simulink model "Loop_Back_Testing"  (R2022a)
settings: Solver=FixedStepAuto  StartTime=0.0  StopTime=inf  FixedStep=.005  RelTol=1e-6
model workspace (MAT data in the model file):
  DEV_ID = 3
libraries: speedgoatlib_IO691 x5, canmsglib x4
settings Model: SimulationMode=external  ExtModeEnableFloating=off  Creator=celwe  LastModifiedBy=celwe
settings SolverCC: ConcurrentTasks=on  PositivePriorityOrder=on
settings OptimizationCC: BlockReduction=off  OptimizeBlockIOStorage=off
settings DebuggingCC: TasksWithSamePriorityMsg=none
settings HardwareCC: ProdBitPerLong=64  ProdLongLongMode=on  ProdHWDeviceType=Intel->x86-64 (Linux 64)
settings RTWCC: Description=Simulink Real-Time  SystemTargetFile=slrealtime.tlc  TemplateMakefile=slrealtime_default_tmf  Toolchain=Simulink Real-Time Toolchain  BuildConfiguration=Faster Runs  CodeExecutionProfiling=on  TargetLang=C++

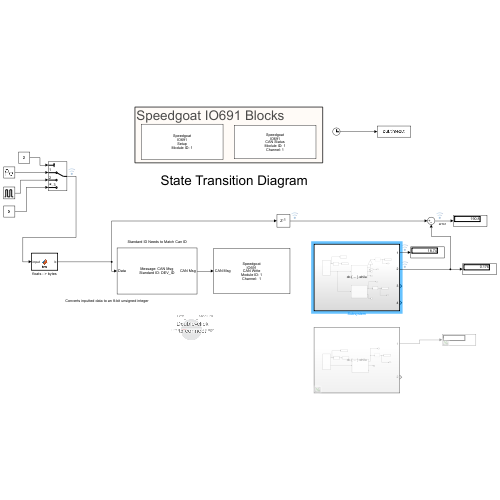
[thumbnail: Simulink's stored preview of the top-level diagram]
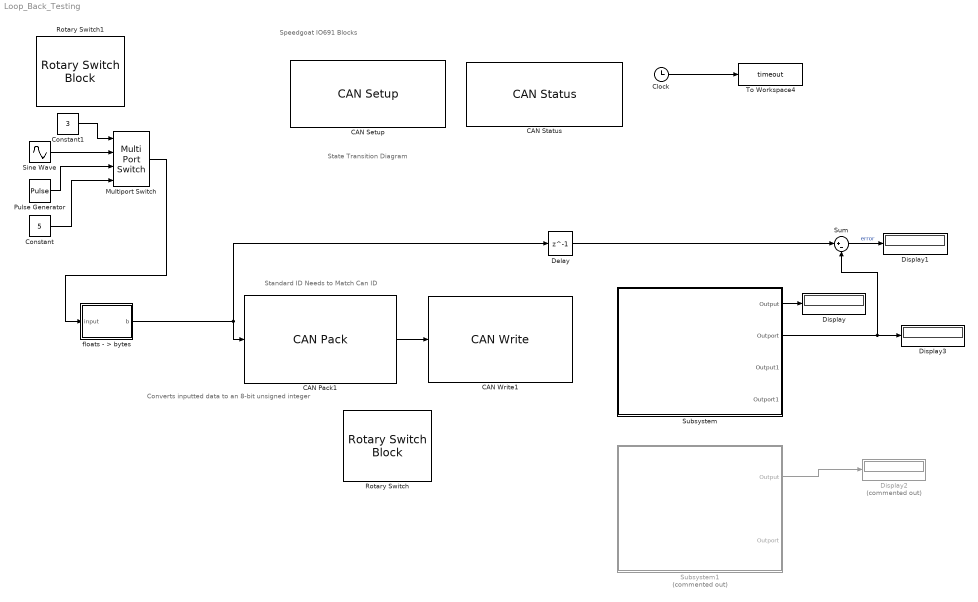
== system Loop_Back_Testing ==
  note: State Transition Diagram
  note: Speedgoat IO691 Blocks
  note: Standard ID Needs to Match Can ID
  note: Converts inputted data to an 8-bit unsigned integer
  CAN Pack1 : canmsglib/CAN Pack  MsgList=(none)  MsgName=CAN Msg  MsgIDType=Standard (11-bit identifier)  MsgIdentifier=DEV_ID  MsgLength=1  Remote=off  ApplyMinMax=off  BusOutput=off  SignalInfo={ 'b1', '0', '8', 'LE', 'unsigned', 'Standard', '0', '1', '0', '-Inf', 'Inf'; 'b2', '8', '8', 'LE', 'unsigned', 'Standard', '0', '1', '0', '-Inf', 'Inf'; 'b3', '16', '8', 'LE', 'unsigned', 'Standard', '0', '1', '0', '-Inf', 'Inf'; 'b4', '24', '8', 'LE', 'unsigned', 'Standard', '0', '1', '0', '-Inf', 'Inf'; 'b5', '32', '8', 'LE', 'unsigned', 'Standard', '0', '1', '0', '-Inf', 'Inf'; 'b6', '40', '8', 'LE', 'unsigned', 'Standard', '0', '1', '0', '-Inf', 'Inf'; 'b7', '48', '8', 'LE', 'unsigned', 'Standard', '0', '1', '0', '-Inf', 'Inf'; 'b8', '56', '8', 'LE', 'unsigned', 'Standard', '0', '1', '0', '-Inf', 'Inf' }
      settings: SourceProductBaseCode=XP,ME,VN  DataFormat=raw data
  "CAN Setup " : speedgoatlib_IO691/Legacy/CAN Setup   moduletype=IO691  id=1  pciSlot=-1  chn1=CAN (HS)  chn2=CAN (HS)  chn3=Disabled  chn4=Disabled  initStruct=[]  termStruct=[]  ArbitrationbdrChn1=1.0 MBaud  ArbitrationManbdrChn1=[2,8,31,8]  FdbdrChn1=5.0 MBaud  FdManbdrChn1=[2,2,5,2]  ArbitrationbdrChn2=1.0 MBaud  ArbitrationManbdrChn2=[2,8,31,8]  FdbdrChn2=5.0 MBaud  FdManbdrChn2=[2,2,5,2]  ArbitrationbdrChn3=1.0 MBaud  ArbitrationManbdrChn3=[2,8,31,8]  FdbdrChn3=5.0 MBaud  FdManbdrChn3=[2,2,5,2]  ArbitrationbdrChn4=1.0 MBaud  ArbitrationManbdrChn4=[2,8,31,8]  FdbdrChn4=5.0 MBaud  FdManbdrChn4=[2,2,5,2]  moduleInitValues=[691 1 -1 -1]
      settings: SourceProductName=Simulink Real-Time: Speedgoat I/O Blockset
  CAN Status : speedgoatlib_IO691/Legacy/CAN Status  moduleId=1  sampleTime=-1  channel=1  busRecovery=Off  arrayOutput=off  controllerCpuLoad=off  controllerLiveCount=off  initModeAct=off  avgBusLoad=off  receiving=off  RxQueueEmpty=off  dataOverrunRcv=off  rxBufferLevel=off  txPending=off  dataOverrunTx=off  txBufferLevel=off  errWarnLimit=off  errPassLimit=off  errBusOff=off  busRecoveryCounter=off  busCouplingErr=off  transceiverErr=off  opMode=off  brp=off  timeSegment1=off  timeSegment2=off  synchronisationJumpWidth=off  dataTSEG1=off  dataTSEG2=off  dataSJW=off  moduleType=691  qtyStatBlk=1  ptIdx=0  isFDMod=0
      settings: SourceProductName=Simulink Real-Time: Speedgoat I/O Blockset
  CAN Write1 : speedgoatlib_IO691/Legacy/CAN Write  id=1  ts=-1  channel=1  messageType=CAN  BusInput=off  enableStatusPort=off  canType=CAN (HS)  initValues=[691 1 -1 0 1 1 0 0]
      settings: SourceProductName=Simulink Real-Time: Speedgoat I/O Blockset
  Clock : Clock
  Constant : Constant  Value=5
  Constant1 : Constant  Value=3
  Delay : Delay  DelayLength=1
  Display : Display
  Display1 : Display
  Display2 : Display  Commented=on
  Display3 : Display
  Multiport Switch : MultiPortSwitch  SaturateOnIntegerOverflow=off  InputSameDT=off
  Pulse Generator : DiscretePulseGenerator  PulseType=Time based  Amplitude=5  Period=5
  Rotary Switch : RotarySwitchBlock
      settings: Values={{'Off', 'Low', 'Medium', 'High'}, [0 1 2 3]}
  Rotary Switch1 : RotarySwitchBlock
      settings: Values={{'Sine Wave', 'Square Wave', 'Constant'}, [1 2 3]}
  Sine Wave : Sin  Amplitude=10  SampleTime=0
  Subsystem : Subsystem
  Subsystem1 : Subsystem  Commented=on
  Sum : Sum  Inputs=|+-
  To Workspace4 : ToWorkspace  VariableName=timeout  SampleTime=-1
  floats - > bytes : MATLAB Function  TreatAsAtomicUnit=on
  wires:
  Clock/1 -> To Workspace4/1
  CAN Pack1/1 -> CAN Write1/1
  floats - > bytes/1(b) -> Delay/1, CAN Pack1/1
  Subsystem/1(Output) -> Display/1
  Multiport Switch/1 -> floats - > bytes/1(input)
  Constant/1 -> Multiport Switch/4
  Pulse Generator/1 -> Multiport Switch/3
  Sum/1 -> Display1/1  "error"
  Subsystem/2(Outport) -> Display3/1, Sum/2
  Delay/1 -> Sum/1
  Subsystem1/1(Output) -> Display2/1
  Constant1/1 -> Multiport Switch/1
  Sine Wave/1 -> Multiport Switch/2

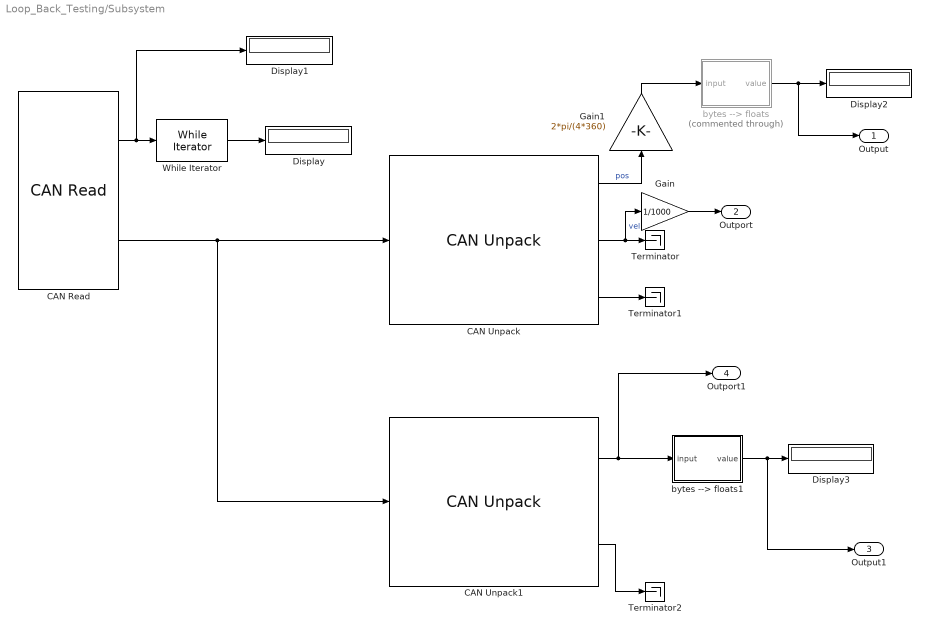
== system Loop_Back_Testing/Subsystem ==
  CAN Read : speedgoatlib_IO691/Legacy/CAN Read  id=1  ts=-1  channel=2  messageType=CAN  canType=CAN (HS)  BusOutput=off  initValues=[691 1 -1 1 1 1 0]
      settings: SourceProductName=Simulink Real-Time: Speedgoat I/O Blockset
  CAN Unpack : canmsglib/CAN Unpack  MsgList=(none)  MsgName=CAN Msg  MsgIDType=Standard (11-bit identifier)  MsgIdentifier=1  MsgLength=6  SignalInfo={ 'pos', '0', '32', 'LE', 'signed', 'Standard', '0', '1', '0', '-Inf', 'Inf'; 'vel', '32', '16', 'LE', 'signed', 'Standard', '0', '1', '0', '-Inf', 'Inf' }  IDPort=off  TimestampPort=off  ErrorPort=off  RemotePort=off  LengthPort=off  StatusPort=on  ApplyMinMax=off
      settings: SourceProductBaseCode=XP,ME,VN
  CAN Unpack1 : canmsglib/CAN Unpack  MsgList=(none)  MsgName=CAN Msg  MsgIDType=Standard (11-bit identifier)  MsgIdentifier=DEV_ID  MsgLength=1  SignalInfo={ 'pos', '0', '8', 'LE', 'signed', 'Standard', '0', '1', '0', '-Inf', 'Inf' }  IDPort=off  TimestampPort=off  ErrorPort=off  RemotePort=off  LengthPort=off  StatusPort=on  ApplyMinMax=off
      settings: SourceProductBaseCode=XP,ME,VN
  Display{,1..3} (4 alike) : Display
  Gain : Gain  Gain=1/1000
  Gain1 : Gain  Gain=2*pi/(4*360)
  Terminator : Terminator
  Terminator1 : Terminator
  Terminator2 : Terminator
  While Iterator : WhileIterator  MaxIters=-1  WhileBlockType=do-while  ResetStates=reset  ShowIterationPort=on
  bytes --> floats : MATLAB Function  Commented=through  TreatAsAtomicUnit=on
  bytes --> floats1 : MATLAB Function  TreatAsAtomicUnit=on
  Output : Outport
  Outport : Outport  Port=2
  Output1 : Outport  Port=3
  Outport1 : Outport  Port=4
  wires:
  CAN Read/1 -> While Iterator/1, Display1/1
  While Iterator/1 -> Display/1
  CAN Unpack/2 -> Gain/1, Terminator/1  "vel"
  CAN Unpack/1 -> Gain1/1  "pos"
  bytes --> floats/1(value) -> Output/1, Display2/1
  CAN Unpack/3 -> Terminator1/1
  CAN Read/2 -> CAN Unpack1/1, CAN Unpack/1
  bytes --> floats1/1(value) -> Output1/1, Display3/1
  CAN Unpack1/2 -> Terminator2/1
  CAN Unpack1/1 -> bytes --> floats1/1(input), Outport1/1
  Gain/1 -> Outport/1
  Gain1/1 -> bytes --> floats/1(input)

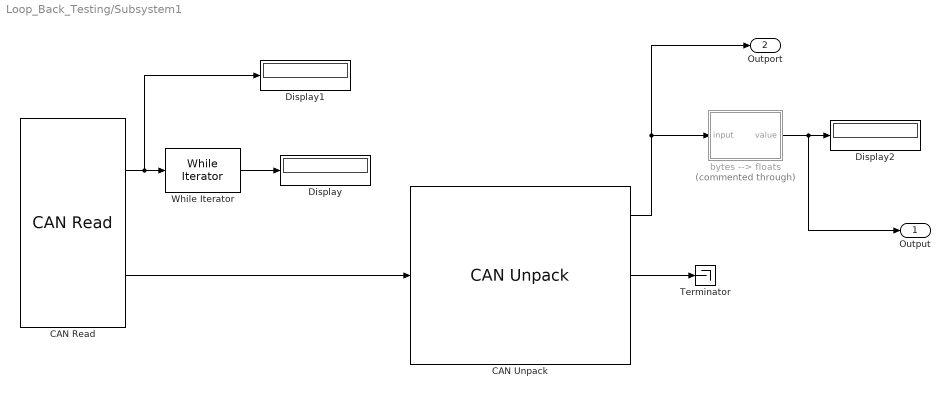
== system Loop_Back_Testing/Subsystem1 ==
  CAN Read : speedgoatlib_IO691/Legacy/CAN Read  id=1  ts=-1  channel=1  messageType=CAN  canType=CAN (HS)  BusOutput=off  initValues=[691 1 -1 0 1 1 0]
      settings: SourceProductName=Simulink Real-Time: Speedgoat I/O Blockset
  CAN Unpack : canmsglib/CAN Unpack  MsgList=(none)  MsgName=CAN Msg  MsgIDType=Standard (11-bit identifier)  MsgIdentifier=2  MsgLength=8  SignalInfo={ 'b1', '0', '8', 'BE', 'unsigned', 'Standard', '0', '1', '0', '-Inf', 'Inf'; 'b2', '8', '8', 'BE', 'unsigned', 'Standard', '0', '1', '0', '-Inf', 'Inf' }  IDPort=off  TimestampPort=off  ErrorPort=off  RemotePort=off  LengthPort=off  StatusPort=on  ApplyMinMax=off
      settings: SourceProductBaseCode=XP,ME,VN
  Display : Display
  Display1 : Display
  Display2 : Display
  Terminator : Terminator
  While Iterator : WhileIterator  MaxIters=-1  WhileBlockType=do-while  ResetStates=reset  ShowIterationPort=on
  bytes --> floats : MATLAB Function  Commented=through  TreatAsAtomicUnit=on
  Output : Outport
  Outport : Outport  Port=2
  wires:
  CAN Read/1 -> While Iterator/1, Display1/1
  While Iterator/1 -> Display/1
  CAN Read/2 -> CAN Unpack/1
  CAN Unpack/2 -> Terminator/1
  CAN Unpack/1 -> bytes --> floats/1(input), Outport/1
  bytes --> floats/1(value) -> Output/1, Display2/1

== matlab function Loop_Back_Testing/floats - > bytes ==
  data: input input; b output
function b = fcn(input)


% P_MIN  =-95.5;  % [rad]
% P_MAX  = 95.5;  % [rad]
input_min = -10;
input_max = 10;

% position = floor((max(min(position,P_MAX) ,P_MIN)  - P_MIN )*65535/(P_MAX  - P_MIN));
value = floor((max(min(input, input_max), input_min) - input_min)*255/(input_max - input_min));

value_bin = dec2bin(value);
%repmat('0', 1, 8-length(value_bin));
value_bin = [repmat('0', 1, 8-length(value_bin)),value_bin];
B = repmat('0', 1, 8);

B(1,:) = value_bin(1:8);

a = bin2dec(B);

b = uint8(a);

== matlab function Loop_Back_Testing/Subsystem1/bytes --> floats ==
  data: input input; value output
function value = fcn(input)

input_min = -10;
input_max = 10;


% P_MIN  =-95.5;  % [rad]
% P_MAX  = 95.5;  % [rad]
% V_MIN  =-45;    % [rad/s]
% V_MAX  = 45;    % [rad/s]
% I_MIN  =-40;    % []
% I_MAX  = 40;    % []

value = double(input)*(input_max - input_min)/255 + input_min;


% position = position*(P_MAX  - P_MIN)/65535+ P_MIN;
% velocity = velocity*(V_MAX  - V_MIN)/4095 + V_MIN;
% I_ff     = I_ff*(I_MAX  - I_MIN)/4095 + I_MIN;

== matlab function Loop_Back_Testing/Subsystem/bytes --> floats1 ==
  data: input input; value output
function value = fcn(input)

input_min = -10;
input_max = 10;


% P_MIN  =-95.5;  % [rad]
% P_MAX  = 95.5;  % [rad]
% V_MIN  =-45;    % [rad/s]
% V_MAX  = 45;    % [rad/s]
% I_MIN  =-40;    % []
% I_MAX  = 40;    % []

value = double(input)*(input_max - input_min)/255 + input_min;


% position = position*(P_MAX  - P_MIN)/65535+ P_MIN;
% velocity = velocity*(V_MAX  - V_MIN)/4095 + V_MIN;
% I_ff     = I_ff*(I_MAX  - I_MIN)/4095 + I_MIN;

== matlab function Loop_Back_Testing/Subsystem/bytes --> floats ==
  data: input input; value output
function value = fcn(input)

input_min = -10;
input_max = 10;


% P_MIN  =-95.5;  % [rad]
% P_MAX  = 95.5;  % [rad]
% V_MIN  =-45;    % [rad/s]
% V_MAX  = 45;    % [rad/s]
% I_MIN  =-40;    % []
% I_MAX  = 40;    % []

value = double(input)*(input_max - input_min)/255 + input_min;


% position = position*(P_MAX  - P_MIN)/65535+ P_MIN;
% velocity = velocity*(V_MAX  - V_MIN)/4095 + V_MIN;
% I_ff     = I_ff*(I_MAX  - I_MIN)/4095 + I_MIN;
